simulink model "Project2_Week2"  (R2023b)
settings: Solver=VariableStepAuto  StartTime=0.0  StopTime=10.0  RelTol=1e-3
settings Model: Creator=vince  LastModifiedBy=vince

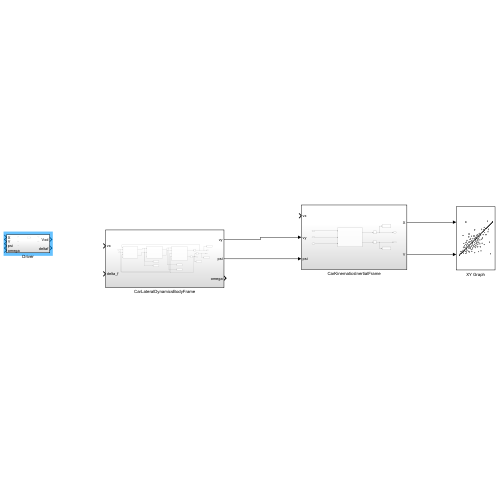
[thumbnail: Simulink's stored preview of the top-level diagram]
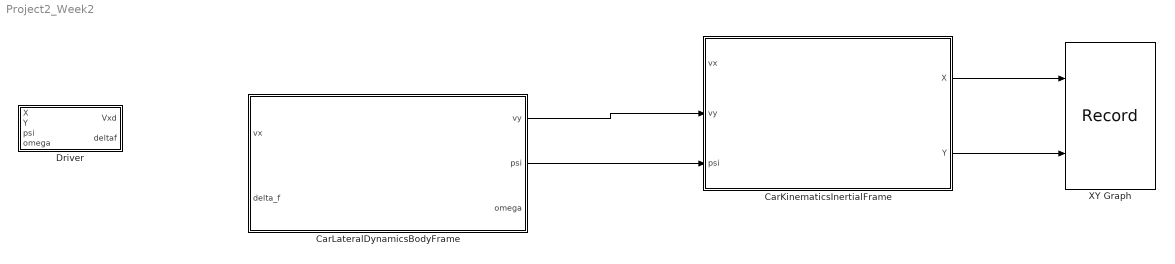
== system Project2_Week2 ==
  CarKinematicsInertialFrame : Subsystem
  CarLateralDynamicsBodyFrame : Subsystem
  Driver : Subsystem
  XY Graph : Record  FileSettingsInternal="{\"entries\":[{\"content\":{\"excelSettings\":{\"content\":{},\"type\":\"Streamout.ExcelSettings\"}},\"type\":\"Streamout.FileSettingStorage\",\"uuid\":\"\"}],\"packageUris\":[\"http:\\/\\/schema.mathworks.com\\/mf0\\/streamout_blocks\\/R2020a\"],\"version\":\"1.0\"}"  Layout=[1 1]  SignalsInternal="{\"entries\":[{\"content\":{\"signals\":[{\"content\":{\"blockPath\":[],\"dimensions\":[1],\"domain\":\"\",\"lineColor\":\"#a2142f\",\"plots\":[1],\"port\":1,\"signalID\":16,\"signalName\":\"XY Graph:1\"},\"type\":\"RecordBlkView.Signal\",\"uuid\":\"\"},{\"content\":{\"blockPath\":[],\"dimensions\":[1],\"domain\":\"\",\"lineColor\":\"#139fff\",\"plots\":[1],\"port\":2,\"signalID\":19,\"signalName\":\"XY Graph:2\"},\"type\":\"RecordBlkView.Signal\",\"uuid\":\"\"}]},\"type\":\"RecordBlkView.InputSignals\",\"uuid\":\"\"}],\"packageUris\":[\"http:\\/\\/schema.mathworks.com\\/mf0\\/streamout_blocks\\/R2020a\"],\"version\":\"1.0\"}"  VisualizationBindings="{\"xyplotplugin\":{\"info\":[{\"series\":[{\"bindingParametersList\":[{\"parameter\":\"X-Axis\",\"signalID\":16,\"signalName\":\"XY Graph:1\"},{\"parameter\":\"Y-Axis\",\"signalID\":19,\"signalName\":\"XY Graph:2\"}],\"seriesID\":19368}],\"subplotID\":1}]}}"  CompatibilityTag=XY
  wires:
  CarKinematicsInertialFrame/1(X) -> XY Graph/1
  CarKinematicsInertialFrame/2(Y) -> XY Graph/2
  CarLateralDynamicsBodyFrame/2(psi) -> CarKinematicsInertialFrame/3(psi)
  CarLateralDynamicsBodyFrame/1(vy) -> CarKinematicsInertialFrame/2(vy)

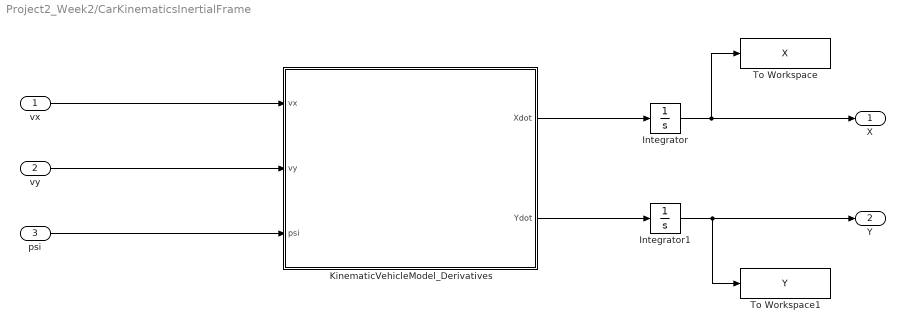
== system Project2_Week2/CarKinematicsInertialFrame ==
  vx : Inport
  vy : Inport  Port=2
  psi : Inport  Port=3
  Integrator : Integrator
  Integrator1 : Integrator
  KinematicVehicleModel_Derivatives : MATLAB Function  TreatAsAtomicUnit=on
  To Workspace : ToWorkspace  VariableName=X  SaveFormat=Timeseries  SampleTime=-1
  To Workspace1 : ToWorkspace  VariableName=Y  SaveFormat=Timeseries  SampleTime=-1
  X : Outport
  Y : Outport  Port=2
  wires:
  vx/1 -> KinematicVehicleModel_Derivatives/1(vx)
  vy/1 -> KinematicVehicleModel_Derivatives/2(vy)
  psi/1 -> KinematicVehicleModel_Derivatives/3(psi)
  KinematicVehicleModel_Derivatives/1(Xdot) -> Integrator/1
  KinematicVehicleModel_Derivatives/2(Ydot) -> Integrator1/1
  Integrator/1 -> To Workspace/1, X/1
  Integrator1/1 -> To Workspace1/1, Y/1

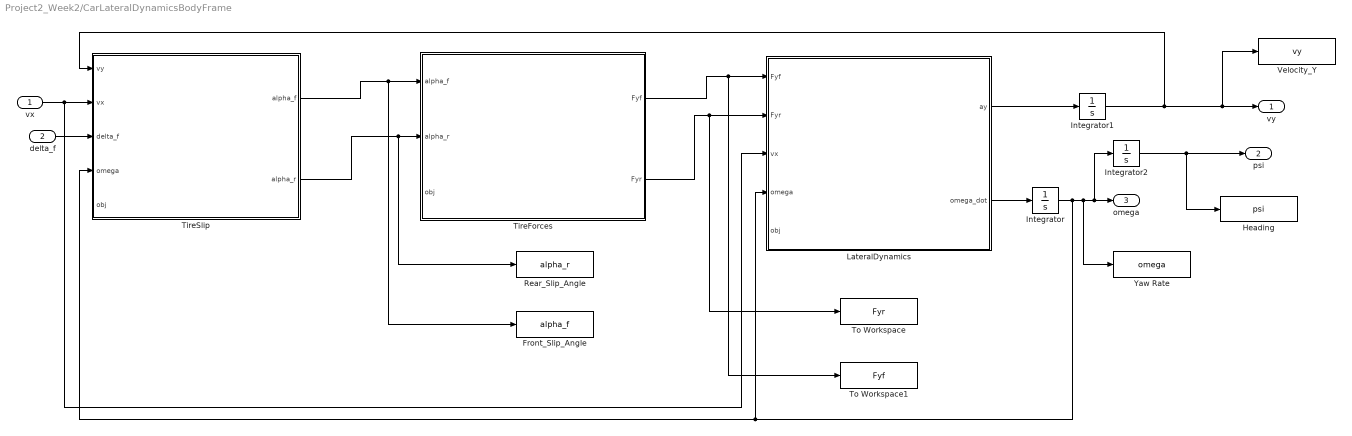
== system Project2_Week2/CarLateralDynamicsBodyFrame ==
  vx : Inport
  delta_f : Inport  Port=2
  Front_Slip_Angle : ToWorkspace  VariableName=alpha_f  SaveFormat=Timeseries  SampleTime=-1
  Heading : ToWorkspace  VariableName=psi  SaveFormat=Timeseries  SampleTime=-1
  Integrator : Integrator
  Integrator1 : Integrator
  Integrator2 : Integrator
  LateralDynamics : MATLAB Function  TreatAsAtomicUnit=on
  Rear_Slip_Angle : ToWorkspace  VariableName=alpha_r  SaveFormat=Timeseries  SampleTime=-1
  TireForces : MATLAB Function  TreatAsAtomicUnit=on
  TireSlip : MATLAB Function  TreatAsAtomicUnit=on
  To Workspace : ToWorkspace  VariableName=Fyr  SaveFormat=Timeseries  SampleTime=-1
  To Workspace1 : ToWorkspace  VariableName=Fyf  SaveFormat=Timeseries  SampleTime=-1
  Velocity_Y : ToWorkspace  VariableName=vy  SaveFormat=Timeseries  SampleTime=-1
  Yaw Rate : ToWorkspace  VariableName=omega  SaveFormat=Timeseries  SampleTime=-1
  vy : Outport
  psi : Outport  Port=2
  omega : Outport  Port=3
  wires:
  delta_f/1 -> TireSlip/3(delta_f)
  TireSlip/2(alpha_r) -> Rear_Slip_Angle/1, TireForces/2(alpha_r)
  TireForces/1(Fyf) -> LateralDynamics/1(Fyf), To Workspace1/1
  TireForces/2(Fyr) -> LateralDynamics/2(Fyr), To Workspace/1
  vx/1 -> TireSlip/2(vx), LateralDynamics/3(vx)
  LateralDynamics/1(ay) -> Integrator1/1
  LateralDynamics/2(omega_dot) -> Integrator/1
  Integrator2/1 -> Heading/1, psi/1
  Integrator1/1 -> TireSlip/1(vy), Velocity_Y/1, vy/1
  Integrator/1 -> LateralDynamics/4(omega), TireSlip/4(omega), Yaw Rate/1, Integrator2/1, omega/1
  TireSlip/1(alpha_f) -> TireForces/1(alpha_f), Front_Slip_Angle/1

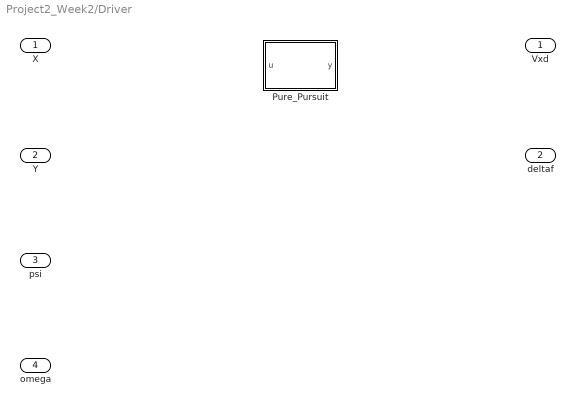
== system Project2_Week2/Driver ==
  X : Inport
  Y : Inport  Port=2
  psi : Inport  Port=3
  omega : Inport  Port=4
  Pure_Pursuit : MATLAB Function  TreatAsAtomicUnit=on
  Vxd : Outport
  deltaf : Outport  Port=2

== matlab function Project2_Week2/CarKinematicsInertialFrame/KinematicVehicleModel_Derivatives ==
  data: vx input; Xdot output; vy input; psi input; Ydot output
function [Xdot, Ydot] = fcn(vx, vy, psi)
    temp = TF(psi) * [vx;vy];
    Xdot = temp(1);
    Ydot = temp(2);
end

function y = TF(psi)
    y = [cos(psi), -sin(psi); sin(psi), cos(psi)];
end

== matlab function Project2_Week2/Driver/Pure_Pursuit ==
  data: u input; y output
function y = fcn(u)

y = u;

== matlab function Project2_Week2/CarLateralDynamicsBodyFrame/TireSlip ==
  data: vy input; alpha_f output; vx input; delta_f input; omega input; obj input; alpha_r output
function [alpha_f, alpha_r] = fnc(vy, vx, delta_f, omega, obj)

    if abs(vx) > obj.vx_threshold1
        alpha_f = delta_f - (vy + omega * obj.lf) / vx;
        alpha_r = - (vy - omega * obj.lr) / vx;
    else
        alpha_f = 0;
        alpha_r = 0;
    end

end

== matlab function Project2_Week2/CarLateralDynamicsBodyFrame/TireForces ==
  data: alpha_f input; Fyf output; alpha_r input; obj input; Fyr output
function [Fyf, Fyr] = fcn(alpha_f, alpha_r, obj)

    Fyf = min(obj.Fyfmax, obj.Calpha_f * alpha_f);
    Fyr = min(obj.Fyrmax, obj.Calpha_r * alpha_r);

end

== matlab function Project2_Week2/CarLateralDynamicsBodyFrame/LateralDynamics ==
  data: Fyf input; ay output; Fyr input; vx input; omega input; obj input; omega_dot output
function [ay, omega_dot] = fcn(Fyf, Fyr, vx, omega, obj)

    Fy = Fyf + Fyr;
    ay = Fy / obj.Mass - omega * vx;

    M = Fyf * obj.lf - Fyr * obj.lr;
    omega_dot = M / obj.Inertia;

end
